simulink model "simmodel"  (R2021b)
settings: Solver=ode4  StartTime=0.0  StopTime=0.001  FixedStep=1e-3  RelTol=1e-3
settings Model: SimulationMode=rapid-accelerator  Creator=valeriytashchilin  LastModifiedBy=valeriytashchilin
settings DataIOCC: InitialState=x  SaveFinalState=on  SaveFormat=Structure  SaveState=on

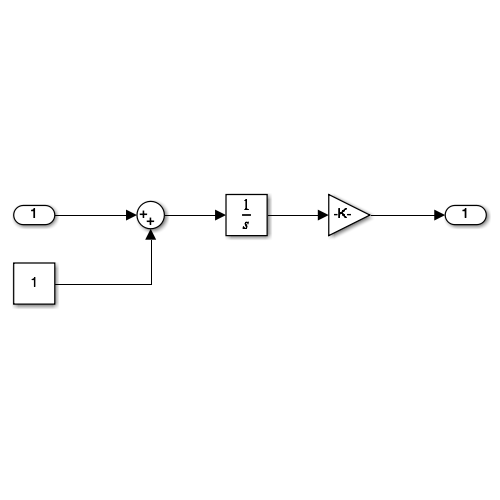
[thumbnail: Simulink's stored preview of the top-level diagram]
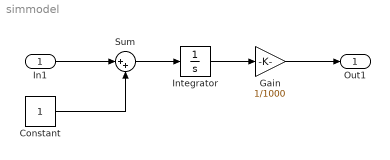
== system simmodel ==
  In1 : Inport
  Constant : Constant
  Gain : Gain  Gain=1/1000
  Integrator : Integrator
  Sum : Sum  Inputs=|++
  Out1 : Outport
  wires:
  In1/1 -> Sum/1
  Constant/1 -> Sum/2
  Sum/1 -> Integrator/1
  Integrator/1 -> Gain/1
  Gain/1 -> Out1/1
